simulink model "control_system"  (R2020b)
settings: Solver=FixedStepAuto  StartTime=0.0  StopTime=t_sim  FixedStep=Ts  RelTol=1e-2
values from neighbouring files (symbols this model uses):
  Hp = 10    [main_script.m]
  InitPosX = -2.4980e+03    (= -2498)    [main_script.m]
  InitPosY = -650.5503    [main_script.m]
  InitVelX = V0*cosd(InitYaw)    [main_script.m]
  InitVelY = V0*sind(InitYaw)    [main_script.m]
  InitYaw = 21    [main_script.m]
  lr = 1.592    [main_script.m]
  m = 1625    [main_script.m]
  Ts = 0.1    [main_script.m]
  V0 = 25    [main_script.m]
libraries: neural x856, simulink x1, autolibshared x1, drivingscenarioandsensors x1
(part 20 of 40)

== system control_system/50 30 1+2+3+14+15+19+22+23+24 curva dx 500m /Layer 3/Delays 1 ==
  "p{3}" : Inport  PortDimensions=30  SampleTime=0.1
      mask Display: e = 0.06;c1 = [120 230 180]/255;c2 = ([120 230 180]+0)/(256+128);c3 = ([120 230 180]+128)/(256+128);patch([0 1 1 0],[0 0 1 1],c1);patch([0 1 1 1-e 1-e 0+e],[0 0 1 1-e 0+e 0+e],c2);patch([0 0 1 1-e 0+e 0+e],[0 1 1 1-e 1-e 0+e],c3);plot([0 1 1 0 0],[0 0 1 1 0]);
  mux : Mux  Inputs=1
      mask Display: e = 0.06;c1 = [120 150 230]/255;c2 = ([120 150 230]+0)/383;c3 = ([120 150 230]+128)/383;patch([0 1 1 0],[0 0 1 1],c1);patch([0 1 1 1-e 1-e 0+e],[0 0 1 1-e 0+e 0+e],c2);patch([0 0 1 1-e 0+e 0+e],[0 1 1 1-e 1-e 0+e],c3);plot([0 1 1 0 0],[0 0 1 1 0]);disp('Mux')
  "pd{3,2}" : Outport
      mask Display: e = 0.06;c1 = [120 230 180]/255;c2 = ([120 230 180]+0)/(256+128);c3 = ([120 230 180]+128)/(256+128);patch([0 1 1 0],[0 0 1 1],c1);patch([0 1 1 1-e 1-e 0+e],[0 0 1 1-e 0+e 0+e],c2);patch([0 0 1 1-e 0+e 0+e],[0 1 1 1-e 1-e 0+e],c3);plot([0 1 1 0 0],[0 0 1 1 0]);
  wires:
  "p{3}"/1 -> mux/1
  mux/1 -> "pd{3,2}"/1

== system control_system/50 30 1+2+3+14+15+19+22+23+24 curva dx 500m /Layer 3/LW{3,2} ==
  "ad{3,2}" : Inport  PortDimensions=30  SampleTime=0.1
      mask Display: e = 0.06;c1 = [120 230 180]/255;c2 = ([120 230 180]+0)/(256+128);c3 = ([120 230 180]+128)/(256+128);patch([0 1 1 0],[0 0 1 1],c1);patch([0 1 1 1-e 1-e 0+e],[0 0 1 1-e 0+e 0+e],c2);patch([0 0 1 1-e 0+e 0+e],[0 1 1 1-e 1-e 0+e],c3);plot([0 1 1 0 0],[0 0 1 1 0]);
  "IW{3,2}(1,:)'" : Constant  Value=[0.274462551045505431801529994118027389049530029296875;0.324672662038586690158581404830329120159149169921875;0.477065195949756770676941641795565374195575714111328125;0.949805854925893644491452505462802946567535400390625;0.300149364011395081153210639968165196478366851806640625;-0.407338902263089941424567541616852395236492156982421875;-0.25072173971622480070919891659286804497241973876953125;1.17952473209077002280764645547606050968170166015625;-1.8869848741233921085580504950485192239284515380859375;0.8473969499470797028806146045099012553691864013671875;-1.2145652621117608571665869021671824157238006591796875;1.30737162436331910697617786354385316371917724609375;0.5862055542077981851178947181324474513530731201171875;-1.1334345562278820285229130604420788586139678955078125;0.347532324809897430473171198173076845705509185791015625;0.454813675484765644885243318640277720987796783447265625;-0.88325051755681316389967605573474429547786712646484375;-0.7616772603757480109010202795616351068019866943359375;-0.1406205812253859266380828785258927382528781890869140625;0.052066530642725809829851613130813348107039928436279296875;1.4716809071902663408337730288621969521045684814453125;0.527725527766693236486617024638690054416656494140625;-0.3145518006265926036491009654127992689609527587890625;-0.62368349512138376855574506407720036804676055908203125;-1.3763266924129056167913631725241430103778839111328125;-0.91717714527678639857555253911414183676242828369140625;-0.99804059332626315903524982786620967090129852294921875;0.2101708948661522857737082858875510282814502716064453125;0.1820155166267572177662970034361933358013629913330078125;-1.9440292881120786461224270169623196125030517578125]
      mask Display: e = 0.06;c1 = [120 150 230]/255;c2 = ([120 150 230]+0)/383;c3 = ([120 150 230]+128)/383;patch([0 1 1 0],[0 0 1 1],c1);patch([0 1 1 1-e 1-e 0+e],[0 0 1 1-e 0+e 0+e],c2);patch([0 0 1 1-e 0+e 0+e],[0 1 1 1-e 1-e 0+e],c3);plot([0 1 1 0 0],[0 0 1 1 0]);disp('weights');
  "IW{3,2}(2,:)'" : Constant  Value=[0.5711243783534591944572866850649006664752960205078125;-0.2447820031055736034186764982223394326865673065185546875;0.71460765933948999784064426421537064015865325927734375;-0.370936768700234453799424727549194358289241790771484375;-0.291045439858436338909086771309375762939453125;-0.038051937430375347426458887412081821821630001068115234375;1.0074294318946641624279436655342578887939453125;-0.6187907564700967366633221899974159896373748779296875;-0.284017344465823773358437165370560251176357269287109375;0.652644060354310884264350534067489206790924072265625;0.6621003571255339448242693833890371024608612060546875;0.2308544894167910699334100854684947989881038665771484375;0.7189141801347418425649493656237609684467315673828125;-0.72567184899621894889065742972888983786106109619140625;-0.162904419463085370356481007547699846327304840087890625;0.27169128301049572105085871953633613884449005126953125;0.17789122131858869924059263212257064878940582275390625;0.354782705810462228868118472746573388576507568359375;0.1664461616962673862207822139680502004921436309814453125;-0.350888605877589021542206637604977004230022430419921875;-0.01400850438531614332304808812068586121313273906707763671875;-0.64196846379309746577490614072303287684917449951171875;0.24504738067695763792386287605040706694126129150390625;0.451748735031426484898275930390809662640094757080078125;-0.45965355672188967783853286164230667054653167724609375;-0.167539227964133285997405664602410979568958282470703125;0.2223229228855519712393373765735304914414882659912109375;-0.221463505478945832383175229551852680742740631103515625;0.59159982562243040860039400286041200160980224609375;-0.217577167130074300427367006705026142299175262451171875]
      mask Display: e = 0.06;c1 = [120 150 230]/255;c2 = ([120 150 230]+0)/383;c3 = ([120 150 230]+128)/383;patch([0 1 1 0],[0 0 1 1],c1);patch([0 1 1 1-e 1-e 0+e],[0 0 1 1-e 0+e 0+e],c2);patch([0 0 1 1-e 0+e 0+e],[0 1 1 1-e 1-e 0+e],c3);plot([0 1 1 0 0],[0 0 1 1 0]);disp('weights');
  Mux : Mux  Inputs=2
      mask Display: e = 0.06;c1 = [120 150 230]/255;c2 = ([120 150 230]+0)/383;c3 = ([120 150 230]+128)/383;patch([0 1 1 0],[0 0 1 1],c1);patch([0 1 1 1-e 1-e 0+e],[0 0 1 1-e 0+e 0+e],c2);patch([0 0 1 1-e 0+e 0+e],[0 1 1 1-e 1-e 0+e],c3);plot([0 1 1 0 0],[0 0 1 1 0]);disp('Mux');
  dotprod1 : neural/Weight Functions/dotprod
  dotprod2 : neural/Weight Functions/dotprod
  "lz{3,2}" : Outport
      mask Display: e = 0.06;c1 = [120 230 180]/255;c2 = ([120 230 180]+0)/(256+128);c3 = ([120 230 180]+128)/(256+128);patch([0 1 1 0],[0 0 1 1],c1);patch([0 1 1 1-e 1-e 0+e],[0 0 1 1-e 0+e 0+e],c2);patch([0 0 1 1-e 0+e 0+e],[0 1 1 1-e 1-e 0+e],c3);plot([0 1 1 0 0],[0 0 1 1 0]);
  wires:
  "IW{3,2}(1,:)'"/1 -> dotprod1/1
  "ad{3,2}"/1 -> dotprod1/2, dotprod2/2
  dotprod1/1 -> Mux/1
  "IW{3,2}(2,:)'"/1 -> dotprod2/1
  dotprod2/1 -> Mux/2
  Mux/1 -> "lz{3,2}"/1

== system control_system/50 30 2+3+4+5+6+7+8+9+16+17 ok rett 100 - 108 /Layer 1/Delays 1 ==
  "p{1}" : Inport  PortDimensions=9  SampleTime=0.1
      mask Display: e = 0.06;c1 = [120 230 180]/255;c2 = ([120 230 180]+0)/(256+128);c3 = ([120 230 180]+128)/(256+128);patch([0 1 1 0],[0 0 1 1],c1);patch([0 1 1 1-e 1-e 0+e],[0 0 1 1-e 0+e 0+e],c2);patch([0 0 1 1-e 0+e 0+e],[0 1 1 1-e 1-e 0+e],c3);plot([0 1 1 0 0],[0 0 1 1 0]);
  mux : Mux  Inputs=1
      mask Display: e = 0.06;c1 = [120 150 230]/255;c2 = ([120 150 230]+0)/383;c3 = ([120 150 230]+128)/383;patch([0 1 1 0],[0 0 1 1],c1);patch([0 1 1 1-e 1-e 0+e],[0 0 1 1-e 0+e 0+e],c2);patch([0 0 1 1-e 0+e 0+e],[0 1 1 1-e 1-e 0+e],c3);plot([0 1 1 0 0],[0 0 1 1 0]);disp('Mux')
  "pd{1,1}" : Outport
      mask Display: e = 0.06;c1 = [120 230 180]/255;c2 = ([120 230 180]+0)/(256+128);c3 = ([120 230 180]+128)/(256+128);patch([0 1 1 0],[0 0 1 1],c1);patch([0 1 1 1-e 1-e 0+e],[0 0 1 1-e 0+e 0+e],c2);patch([0 0 1 1-e 0+e 0+e],[0 1 1 1-e 1-e 0+e],c3);plot([0 1 1 0 0],[0 0 1 1 0]);
  wires:
  "p{1}"/1 -> mux/1
  mux/1 -> "pd{1,1}"/1
